simulink model "motion_sim"  (R2020a)
settings: Solver=ode4  StartTime=0.0  StopTime=20  FixedStep=Tc  RelTol=1e-3
values from neighbouring files (symbols this model uses):
  vx_ini = 30    [para_set.m]
  vy_ini = 0    [para_set.m]
  X_ini = 0    [para_set.m]
  Y_ini = 0    [para_set.m]
  yaw_ini = 0    [para_set.m]
  yawrate_ini = 0    [para_set.m]
undefined symbols (not defined in the file or in its folder): global_motion, vehicle_motion, vehicle_motion_nonlinear
settings Model: Creator=Mook  LastModifiedBy=Mook
settings DataIOCC: ReturnWorkspaceOutputs=off

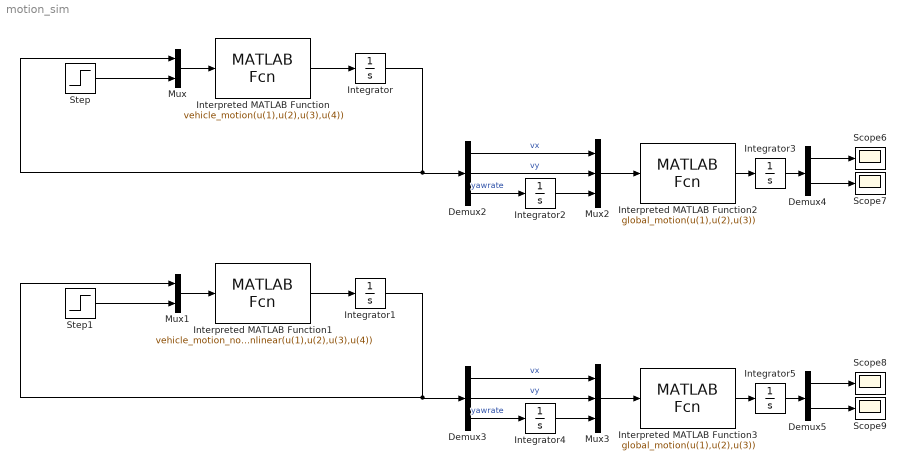
== system motion_sim ==
  Demux2 : Demux  Outputs=3
  Demux3 : Demux  Outputs=3
  Demux4 : Demux  Outputs=2
  Demux5 : Demux  Outputs=2
  Integrator : Integrator  InitialCondition=[vx_ini; vy_ini; yawrate_ini]
  Integrator1 : Integrator  InitialCondition=[vx_ini vy_ini yawrate_ini]
  Integrator2 : Integrator  InitialCondition=[yaw_ini]
  Integrator3 : Integrator  InitialCondition=[X_ini Y_ini]
  Integrator4 : Integrator  InitialCondition=[yaw_ini]
  Integrator5 : Integrator  InitialCondition=[X_ini Y_ini]
  Interpreted MATLAB Function : MATLABFcn  MATLABFcn=vehicle_motion(u(1),u(2),u(3),u(4))  OutputDimensions=3
  Interpreted MATLAB Function1 : MATLABFcn  MATLABFcn=vehicle_motion_nonlinear(u(1),u(2),u(3),u(4))  OutputDimensions=3
  Interpreted MATLAB Function2 : MATLABFcn  MATLABFcn=global_motion(u(1),u(2),u(3))  OutputDimensions=2
  Interpreted MATLAB Function3 : MATLABFcn  MATLABFcn=global_motion(u(1),u(2),u(3))  OutputDimensions=2
  Mux : Mux  Inputs=2
  Mux1 : Mux  Inputs=2
  Mux2 : Mux  Inputs=3
  Mux3 : Mux  Inputs=3
  Scope{6..9} (4 alike) : Scope
  Step : Step  Time=2  After=10*pi/180  SampleTime=0
  Step1 : Step  Time=2  After=10*pi/180  SampleTime=0
  wires:
  Mux/1 -> Interpreted MATLAB Function/1
  Interpreted MATLAB Function/1 -> Integrator/1
  Integrator/1 -> Demux2/1, Mux/1
  Step/1 -> Mux/2
  Interpreted MATLAB Function1/1 -> Integrator1/1
  Integrator1/1 -> Demux3/1, Mux1/1
  Mux1/1 -> Interpreted MATLAB Function1/1
  Step1/1 -> Mux1/2
  Demux2/3 -> Integrator2/1  "yawrate"
  Integrator2/1 -> Mux2/3
  Demux2/2 -> Mux2/2  "vy"
  Demux2/1 -> Mux2/1  "vx"
  Mux2/1 -> Interpreted MATLAB Function2/1
  Interpreted MATLAB Function2/1 -> Integrator3/1
  Integrator3/1 -> Demux4/1
  Demux3/3 -> Integrator4/1  "yawrate"
  Mux3/1 -> Interpreted MATLAB Function3/1
  Demux3/1 -> Mux3/1  "vx"
  Integrator5/1 -> Demux5/1
  Integrator4/1 -> Mux3/3
  Interpreted MATLAB Function3/1 -> Integrator5/1
  Demux3/2 -> Mux3/2  "vy"
  Demux4/1 -> Scope6/1
  Demux4/2 -> Scope7/1
  Demux5/1 -> Scope8/1
  Demux5/2 -> Scope9/1
